simulink model "CF018A_GmRoadWhlInQlfr"  (R2013b)
settings: Solver=FixedStepDiscrete  SolverMode=SingleTasking  StartTime=0.0  StopTime=1  FixedStep=0.002  RelTol=1e-3
values from neighbouring files (symbols this model uses):
  DELTAPLSROLLOVR_CNT_S16 = DataDict.Constant    [CF018A_GmRoadWhlInQlfr_DataDict.m]
  DELTATISTAMPCNTROLLOVR_CNT_S32 = DataDict.Constant    [CF018A_GmRoadWhlInQlfr_DataDict.m]
  GmRoadWhlInQlfrMaxAllwblFrq = DataDict.Calibration    [CF018A_GmRoadWhlInQlfr_DataDict.m]
  GmRoadWhlInQlfrMaxFrqChg = DataDict.Calibration    [CF018A_GmRoadWhlInQlfr_DataDict.m]
  LEFRQCHGOUTOFRNG_CNT_U08 = DataDict.Constant    [CF018A_GmRoadWhlInQlfr_DataDict.m]
  LEFRQOUTOFRNG_CNT_U08 = DataDict.Constant    [CF018A_GmRoadWhlInQlfr_DataDict.m]
  NODEBSTEP_CNT_U16 = DataDict.Constant    [CF018A_GmRoadWhlInQlfr_DataDict.m]
  PARKDURN_CNT_F32 = DataDict.Constant    [CF018A_GmRoadWhlInQlfr_DataDict.m]
  PREVRAWWHLFRQMIN_HZ_F32 = DataDict.Constant    [CF018A_GmRoadWhlInQlfr_DataDict.m]
  RIFRQCHGOUTOFRNG_CNT_U08 = DataDict.Constant    [CF018A_GmRoadWhlInQlfr_DataDict.m]
  RIFRQOUTOFRNG_CNT_U08 = DataDict.Constant    [CF018A_GmRoadWhlInQlfr_DataDict.m]
  SECTO100MICROSECCNVN_CNT_F32 = DataDict.Constant    [CF018A_GmRoadWhlInQlfr_DataDict.m]
  WHLFRQMIN_HZ_F32 = DataDict.Constant    [CF018A_GmRoadWhlInQlfr_DataDict.m]
undefined symbols (not defined in the file or in its folder): NtcNr1, NtcSts1
libraries: simulink x8, NxtrAbslt x2, NxtrLim x2
(part 2 of 5)

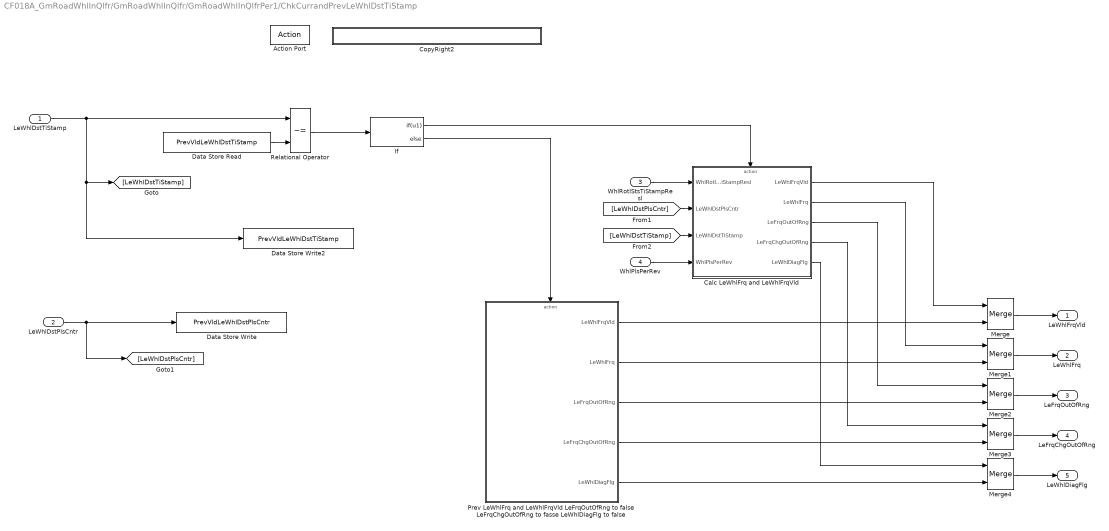
== system CF018A_GmRoadWhlInQlfr/GmRoadWhlInQlfr/GmRoadWhlInQlfrPer1/ChkCurrandPrevLeWhlDstTiStamp ==
  LeWhlDstTiStamp : Inport  RequirementInfo="{'linktype_rmi_doors' '0000c6e7 (/GM T1XX/SubSystem Specifications/Customer Functions/CF018A GM Road Wheel Input Qualifier)' '#174' 'true' 'REQ:  174' '' ; 'linktype_rmi_doors' '0000c6e7 (/GM T1XX/SubSystem Specifications/Customer Functions/CF018A GM Road Wheel Input Qualifier)' '#172' 'true' 'REQ:  172' '' ; 'linktype_rmi_doors' '0000c6e7 (/GM T1XX/SubSystem Specifications/Customer Functions/CF018A GM Road Wheel Input Qualifier)' '#172' 'true' 'REQ:  172' '' } %GIDa_1edc5147_117f_466a_8f92_e1f300aba7a4"
  LeWhlDstPlsCntr : Inport  RequirementInfo="{'linktype_rmi_doors' '0000c6e7 (/GM T1XX/SubSystem Specifications/Customer Functions/CF018A GM Road Wheel Input Qualifier)' '#174' 'true' 'REQ:  174' '' ; 'linktype_rmi_doors' '0000c6e7 (/GM T1XX/SubSystem Specifications/Customer Functions/CF018A GM Road Wheel Input Qualifier)' '#172' 'true' 'REQ:  172' '' } %GIDa_599ac311_8a22_418b_b4e0_03b5bb744075"  Port=2
  WhlRotlStsTiStampResl : Inport  RequirementInfo="{'linktype_rmi_doors' '0000c6e7 (/GM T1XX/SubSystem Specifications/Customer Functions/CF018A GM Road Wheel Input Qualifier)' '#172' 'true' 'REQ:  172' '' } %GIDa_a6510751_6b9d_4ed4_a7a9_c0455e316efd"  Port=3
  WhlPlsPerRev : Inport  RequirementInfo="{'linktype_rmi_doors' '0000c6e7 (/GM T1XX/SubSystem Specifications/Customer Functions/CF018A GM Road Wheel Input Qualifier)' '#172' 'true' 'REQ:  172' '' } %GIDa_b7be02b7_11d7_40a6_809e_b2017e30a38a"  Port=4
  Action Port : ActionPort  ActionType=else
  "Calc LeWhlFrq and LeWhlFrqVld " : Subsystem  RequirementInfo="{'linktype_rmi_doors' '0000c6e7 (/GM T1XX/SubSystem Specifications/Customer Functions/CF018A GM Road Wheel Input Qualifier)' '#172' 'true' 'REQ:  172' '' } %GIDa_4f3dc1f5_4afb_4260_bb3a_586610af36fa"  TreatAsAtomicUnit=on
      settings: AttributesFormatString=%<Priority>
  CopyRight2 : Subsystem  Description=|  mask(Copyright Information){none=on}
      | Copyright info block.                                               
      |                                                                     
      | Place copyright information at the top of every subsystem in design.
      mask prompts: none "No parameters"
      mask help: Place copyright information at the top of every subsystem in design.
      mask Display:
      | NxtrConf = 'Nexteer Confidential';
      | 
      | sys = bdroot; %handle for the current model ("system")
      | first = get_param(sys,'Created');
      | if(isempty(first))
      |     first = datestr(now,'yyyy');
      | else
      |     first = first(end-3:end);  %year is last four digits
      | end
      | 
      | last = get_param(sys,'LastModifiedDate');
      | if isempty(last)
      |     last = datestr(now,'yyyy');
      | else
      |     last = last(end-3:end);
      | end
      | 
      | if strcmp(first,last)
      |     fprintf('%s -- Copyright %s Nexteer',NxtrConf,first)
      | else
      |     fprintf('%s -- %s%s- %s Nexteer',NxtrConf,char(169),first,last)
      | end
  Data Store Read : DataStoreRead  RequirementInfo="{'linktype_rmi_doors' '0000c6e7 (/GM T1XX/SubSystem Specifications/Customer Functions/CF018A GM Road Wheel Input Qualifier)' '#174' 'true' 'REQ:  174' '' ; 'linktype_rmi_doors' '0000c6e7 (/GM T1XX/SubSystem Specifications/Customer Functions/CF018A GM Road Wheel Input Qualifier)' '#172' 'true' 'REQ:  172' '' ; 'linktype_rmi_doors' '0000c6e7 (/GM T1XX/SubSystem Specifications/Customer Functions/CF018A GM Road Wheel Input Qualifier)' '#172' 'true' 'REQ:  172' '' } %GIDa_b02de942_6a04_4580_afa9_b3288210702f"  Priority=0  DataStoreName=PrevVldLeWhlDstTiStamp
      settings: AttributesFormatString=%<Priority>
  Data Store Write : DataStoreWrite  RequirementInfo="{'linktype_rmi_doors' '0000c6e7 (/GM T1XX/SubSystem Specifications/Customer Functions/CF018A GM Road Wheel Input Qualifier)' '#174' 'true' 'REQ:  174' '' ; 'linktype_rmi_doors' '0000c6e7 (/GM T1XX/SubSystem Specifications/Customer Functions/CF018A GM Road Wheel Input Qualifier)' '#172' 'true' 'REQ:  172' '' } %GIDa_a502ae3f_c815_4164_88b0_c5b442c65c19"  Priority=2  DataStoreName=PrevVldLeWhlDstPlsCntr
      settings: AttributesFormatString=%<Priority>
  Data Store Write2 : DataStoreWrite  RequirementInfo="{'linktype_rmi_doors' '0000c6e7 (/GM T1XX/SubSystem Specifications/Customer Functions/CF018A GM Road Wheel Input Qualifier)' '#174' 'true' 'REQ:  174' '' ; 'linktype_rmi_doors' '0000c6e7 (/GM T1XX/SubSystem Specifications/Customer Functions/CF018A GM Road Wheel Input Qualifier)' '#172' 'true' 'REQ:  172' '' } %GIDa_ece9e0a0_953f_437a_8e6e_b4cc8c21fda4"  Priority=2  DataStoreName=PrevVldLeWhlDstTiStamp
      settings: AttributesFormatString=%<Priority>
  If : If  RequirementInfo="{'linktype_rmi_doors' '0000c6e7 (/GM T1XX/SubSystem Specifications/Customer Functions/CF018A GM Road Wheel Input Qualifier)' '#174' 'true' 'REQ:  174' '' ; 'linktype_rmi_doors' '0000c6e7 (/GM T1XX/SubSystem Specifications/Customer Functions/CF018A GM Road Wheel Input Qualifier)' '#172' 'true' 'REQ:  172' '' ; 'linktype_rmi_doors' '0000c6e7 (/GM T1XX/SubSystem Specifications/Customer Functions/CF018A GM Road Wheel Input Qualifier)' '#172' 'true' 'REQ:  172' '' } %GIDa_623ca339_0f35_4816_a941_00824c8527d2"  Priority=1  IfExpression=u1
      settings: AttributesFormatString=%<Priority>
  Merge{,1..4} (5 alike) : Merge
  "Prev LeWhlFrq and LeWhlFrqVld LeFrqOutOfRng to false LeFrqChgOutOfRng to fasse LeWhlDiagFlg to false " : Subsystem  RequirementInfo="{'linktype_rmi_doors' '0000c6e7 (/GM T1XX/SubSystem Specifications/Customer Functions/CF018A GM Road Wheel Input Qualifier)' '#174' 'true' 'REQ:  174' '' } %GIDa_5ebd6336_ff2e_47bd_9598_9199716c73c5"  TreatAsAtomicUnit=on
  Relational Operator : RelationalOperator  RequirementInfo="{'linktype_rmi_doors' '0000c6e7 (/GM T1XX/SubSystem Specifications/Customer Functions/CF018A GM Road Wheel Input Qualifier)' '#174' 'true' 'REQ:  174' '' ; 'linktype_rmi_doors' '0000c6e7 (/GM T1XX/SubSystem Specifications/Customer Functions/CF018A GM Road Wheel Input Qualifier)' '#172' 'true' 'REQ:  172' '' ; 'linktype_rmi_doors' '0000c6e7 (/GM T1XX/SubSystem Specifications/Customer Functions/CF018A GM Road Wheel Input Qualifier)' '#172' 'true' 'REQ:  172' '' } %GIDa_87ebce60_f387_4632_9316_04e7de82df91"  Operator=~=  OutDataTypeStr=boolean
  LeWhlFrqVld : Outport
  LeWhlFrq : Outport  Port=2
  LeFrqOutOfRng : Outport  Port=3
  LeFrqChgOutOfRng : Outport  Port=4
  LeWhlDiagFlg : Outport  Port=5
  wires:
  If/1 -> "Calc LeWhlFrq and LeWhlFrqVld "/Action
  WhlRotlStsTiStampResl/1 -> "Calc LeWhlFrq and LeWhlFrqVld "/1(WhlRotlStsTiStampResl)
  LeWhlDstPlsCntr/1 -> Data Store Write/1, [LeWhlDstPlsCntr]
  [LeWhlDstPlsCntr] -> "Calc LeWhlFrq and LeWhlFrqVld "/2(LeWhlDstPlsCntr)
  [LeWhlDstTiStamp] -> "Calc LeWhlFrq and LeWhlFrqVld "/3(LeWhlDstTiStamp)
  WhlPlsPerRev/1 -> "Calc LeWhlFrq and LeWhlFrqVld "/4(WhlPlsPerRev)
  Relational Operator/1 -> If/1
  Data Store Read/1 -> Relational Operator/2
  LeWhlDstTiStamp/1 -> Relational Operator/1, Data Store Write2/1, [LeWhlDstTiStamp]
  If/2 -> "Prev LeWhlFrq and LeWhlFrqVld LeFrqOutOfRng to false LeFrqChgOutOfRng to fasse LeWhlDiagFlg to false "/Action
  "Prev LeWhlFrq and LeWhlFrqVld LeFrqOutOfRng to false LeFrqChgOutOfRng to fasse LeWhlDiagFlg to false "/4(LeFrqChgOutOfRng) -> Merge3/2
  "Prev LeWhlFrq and LeWhlFrqVld LeFrqOutOfRng to false LeFrqChgOutOfRng to fasse LeWhlDiagFlg to false "/3(LeFrqOutOfRng) -> Merge2/2
  "Prev LeWhlFrq and LeWhlFrqVld LeFrqOutOfRng to false LeFrqChgOutOfRng to fasse LeWhlDiagFlg to false "/2(LeWhlFrq) -> Merge1/2
  "Prev LeWhlFrq and LeWhlFrqVld LeFrqOutOfRng to false LeFrqChgOutOfRng to fasse LeWhlDiagFlg to false "/1(LeWhlFrqVld) -> Merge/2
  "Calc LeWhlFrq and LeWhlFrqVld "/1(LeWhlFrqVld) -> Merge/1
  "Calc LeWhlFrq and LeWhlFrqVld "/2(LeWhlFrq) -> Merge1/1
  "Calc LeWhlFrq and LeWhlFrqVld "/3(LeFrqOutOfRng) -> Merge2/1
  "Calc LeWhlFrq and LeWhlFrqVld "/4(LeFrqChgOutOfRng) -> Merge3/1
  Merge/1 -> LeWhlFrqVld/1
  Merge1/1 -> LeWhlFrq/1
  Merge2/1 -> LeFrqOutOfRng/1
  Merge3/1 -> LeFrqChgOutOfRng/1
  "Calc LeWhlFrq and LeWhlFrqVld "/5(LeWhlDiagFlg) -> Merge4/1
  "Prev LeWhlFrq and LeWhlFrqVld LeFrqOutOfRng to false LeFrqChgOutOfRng to fasse LeWhlDiagFlg to false "/5(LeWhlDiagFlg) -> Merge4/2
  Merge4/1 -> LeWhlDiagFlg/1

== system CF018A_GmRoadWhlInQlfr/GmRoadWhlInQlfr/GmRoadWhlInQlfrPer1/CopyRight2 ==

== system CF018A_GmRoadWhlInQlfr/GmRoadWhlInQlfr/GmRoadWhlInQlfrPer1/NTC Diag ==
  LeFrqOutOfRng : Inport  RequirementInfo="{'linktype_rmi_doors' '0000c6e7 (/GM T1XX/SubSystem Specifications/Customer Functions/CF018A GM Road Wheel Input Qualifier)' '#53' 'true' 'REQ:  53' '' } %GIDa_bae70605_31ad_47de_93e2_34b5a485cde8"
  LeFrqChgOutOfRng : Inport  RequirementInfo="{'linktype_rmi_doors' '0000c6e7 (/GM T1XX/SubSystem Specifications/Customer Functions/CF018A GM Road Wheel Input Qualifier)' '#53' 'true' 'REQ:  53' '' } %GIDa_e1b25c35_a3b3_48ae_865c_0be9f62ee40d"  Port=2
  RiFrqOutOfRng : Inport  RequirementInfo="{'linktype_rmi_doors' '0000c6e7 (/GM T1XX/SubSystem Specifications/Customer Functions/CF018A GM Road Wheel Input Qualifier)' '#53' 'true' 'REQ:  53' '' } %GIDa_31ff7ea8_be27_4839_9d0c_e89098cdec37"  Port=3
  RiFrqChgOutOfRng : Inport  RequirementInfo="{'linktype_rmi_doors' '0000c6e7 (/GM T1XX/SubSystem Specifications/Customer Functions/CF018A GM Road Wheel Input Qualifier)' '#53' 'true' 'REQ:  53' '' } %GIDa_d26123b2_819a_4208_b0a7_2d9f46403555"  Port=4
  Action Port : ActionPort  ActionType=then
  Constant7 : Constant  RequirementInfo="{'linktype_rmi_doors' '0000c6e7 (/GM T1XX/SubSystem Specifications/Customer Functions/CF018A GM Road Wheel Input Qualifier)' '#53' 'true' 'REQ:  53' '' } %GIDa_40ab3d2e_6992_4126_9d67_b6070ef67c87"  Value=NODEBSTEP_CNT_U16
  Constant8 : Constant  RequirementInfo="{'linktype_rmi_doors' '0000c6e7 (/GM T1XX/SubSystem Specifications/Customer Functions/CF018A GM Road Wheel Input Qualifier)' '#53' 'true' 'REQ:  53' '' } %GIDa_77dfdcf3_e931_43d1_8caf_f6541dba129c"  Value=0  OutDataTypeStr=uint8
  Enumerated Constant2 : simulink/Sources/Enumerated Constant  RequirementInfo="{'linktype_rmi_doors' '0000c6e7 (/GM T1XX/SubSystem Specifications/Customer Functions/CF018A GM Road Wheel Input Qualifier)' '#53' 'true' 'REQ:  53' '' } %GIDa_ff40414a_bc98_44c9_a836_28923ef7b0e2"  OutDataTypeStr=Enum: NtcNr1  Value=NtcNr1.NTCNR_0X0E3  SampleTime=inf
  Enumerated Constant3 : simulink/Sources/Enumerated Constant  RequirementInfo="{'linktype_rmi_doors' '0000c6e7 (/GM T1XX/SubSystem Specifications/Customer Functions/CF018A GM Road Wheel Input Qualifier)' '#53' 'true' 'REQ:  53' '' } %GIDa_cfcf815d_81ef_4798_a053_4d41e7c75542"  OutDataTypeStr=Enum: NtcSts1  Value=NtcSts1.NTCSTS_PASSD  SampleTime=inf
  If2 : If  RequirementInfo="{'linktype_rmi_doors' '0000c6e7 (/GM T1XX/SubSystem Specifications/Customer Functions/CF018A GM Road Wheel Input Qualifier)' '#53' 'true' 'REQ:  53' '' } %GIDa_3353ee46_94e0_40a5_b784_e082bbbbc02d"  IfExpression=u1
  Logical Operator : Logic  RequirementInfo="{'linktype_rmi_doors' '0000c6e7 (/GM T1XX/SubSystem Specifications/Customer Functions/CF018A GM Road Wheel Input Qualifier)' '#53' 'true' 'REQ:  53' '' } %GIDa_fa2d2b95_4496_42fd_8f91_86f1fb2eadd8"  Operator=OR  Inputs=4  AllPortsSameDT=off  OutDataTypeStr=boolean
  NTC 0x0E3 Faild : Subsystem  RequirementInfo="{'linktype_rmi_doors' '0000c6e7 (/GM T1XX/SubSystem Specifications/Customer Functions/CF018A GM Road Wheel Input Qualifier)' '#53' 'true' 'REQ:  53' '' } %GIDa_49e1fe86_dba3_482d_9812_54f10c7cfaaf"  TreatAsAtomicUnit=on
  NTC 0x0E3 Passd : Subsystem  RequirementInfo="{'linktype_rmi_doors' '0000c6e7 (/GM T1XX/SubSystem Specifications/Customer Functions/CF018A GM Road Wheel Input Qualifier)' '#53' 'true' 'REQ:  53' '' } %GIDa_3990bfa5_7e5f_4316_8018_426f321c385b"  mask(SetNTC){}
      mask help: SetNTC library block
  wires:
  Logical Operator/1 -> If2/1
  If2/1 -> NTC 0x0E3 Faild/Action
  If2/2 -> NTC 0x0E3 Passd/Action
  Enumerated Constant2/1 -> NTC 0x0E3 Passd/1(NtcNr)
  Enumerated Constant3/1 -> NTC 0x0E3 Passd/3(NtcSts)
  Constant7/1 -> NTC 0x0E3 Passd/4(DebStep)
  Constant8/1 -> NTC 0x0E3 Passd/2(NtcStInfo)
  LeFrqOutOfRng/1 -> NTC 0x0E3 Faild/1(LeFrqOutOfRng), Logical Operator/1
  LeFrqChgOutOfRng/1 -> NTC 0x0E3 Faild/2(LeFrqChgOutOfRng), Logical Operator/2
  RiFrqOutOfRng/1 -> NTC 0x0E3 Faild/3(RiFrqOutOfRng), Logical Operator/3
  RiFrqChgOutOfRng/1 -> NTC 0x0E3 Faild/4(RiFrqChgOutOfRng), Logical Operator/4

== system CF018A_GmRoadWhlInQlfr/GmRoadWhlInQlfr/GmRoadWhlInQlfrPer1/Set Min Le whl Frq and false  ==
  Action Port : ActionPort  ActionType=then
  Constant1 : Constant  Value=WHLFRQMIN_HZ_F32  OutDataTypeStr=single
  Constant2 : Constant  Value=false  OutDataTypeStr=boolean
      settings: AttributesFormatString=%<OutDataTypeStr>
  CopyRight2 : Subsystem  Description=|  mask(Copyright Information){none=on}
      | Copyright info block.                                               
      |                                                                     
      | Place copyright information at the top of every subsystem in design.
      mask prompts: none "No parameters"
      mask help: Place copyright information at the top of every subsystem in design.
      mask Display:
      | NxtrConf = 'Nexteer Confidential';
      | 
      | sys = bdroot; %handle for the current model ("system")
      | first = get_param(sys,'Created');
      | if(isempty(first))
      |     first = datestr(now,'yyyy');
      | else
      |     first = first(end-3:end);  %year is last four digits
      | end
      | 
      | last = get_param(sys,'LastModifiedDate');
      | if isempty(last)
      |     last = datestr(now,'yyyy');
      | else
      |     last = last(end-3:end);
      | end
      | 
      | if strcmp(first,last)
      |     fprintf('%s -- Copyright %s Nexteer',NxtrConf,first)
      | else
      |     fprintf('%s -- %s%s- %s Nexteer',NxtrConf,char(169),first,last)
      | end
  LeWhlFrqVld : Outport
  LeWhlFrq : Outport  Port=2
  wires:
  Constant1/1 -> LeWhlFrq/1
  Constant2/1 -> LeWhlFrqVld/1

== system CF018A_GmRoadWhlInQlfr/GmRoadWhlInQlfr/GmRoadWhlInQlfrPer1/Set Min Ri whl Frq and false  ==
  Action Port : ActionPort  ActionType=then
  Constant1 : Constant  Value=WHLFRQMIN_HZ_F32  OutDataTypeStr=single
  Constant2 : Constant  Value=false  OutDataTypeStr=boolean
      settings: AttributesFormatString=%<OutDataTypeStr>
  CopyRight2 : Subsystem  Description=|  mask(Copyright Information){none=on}
      | Copyright info block.                                               
      |                                                                     
      | Place copyright information at the top of every subsystem in design.
      mask prompts: none "No parameters"
      mask help: Place copyright information at the top of every subsystem in design.
      mask Display:
      | NxtrConf = 'Nexteer Confidential';
      | 
      | sys = bdroot; %handle for the current model ("system")
      | first = get_param(sys,'Created');
      | if(isempty(first))
      |     first = datestr(now,'yyyy');
      | else
      |     first = first(end-3:end);  %year is last four digits
      | end
      | 
      | last = get_param(sys,'LastModifiedDate');
      | if isempty(last)
      |     last = datestr(now,'yyyy');
      | else
      |     last = last(end-3:end);
      | end
      | 
      | if strcmp(first,last)
      |     fprintf('%s -- Copyright %s Nexteer',NxtrConf,first)
      | else
      |     fprintf('%s -- %s%s- %s Nexteer',NxtrConf,char(169),first,last)
      | end
  RiWhlFrqVld : Outport
  RiWhlFrq : Outport  Port=2
  wires:
  Constant2/1 -> RiWhlFrqVld/1
  Constant1/1 -> RiWhlFrq/1

== system CF018A_GmRoadWhlInQlfr/GmRoadWhlInQlfr/GmRoadWhlInQlfrInit1/NTC 0x0E3 Passd/SetNtcSts ==
  NtcNr : Inport
  NtcStInfo : Inport  Port=2
  NtcSts : Inport  Port=3
  DebStep : Inport  Port=4
  CopyRight2 : Subsystem  Description=|  mask(Copyright Information){none=on}
      | Copyright info block.                                               
      |                                                                     
      | Place copyright information at the top of every subsystem in design.
      mask prompts: none "No parameters"
      mask help: Place copyright information at the top of every subsystem in design.
      mask Display:
      | NxtrConf = 'Nexteer Confidential';
      | 
      | sys = bdroot; %handle for the current model ("system")
      | first = get_param(sys,'Created');
      | first = first(end-3:end);  %year is last four digits
      | 
      | last = get_param(sys,'LastModifiedDate');
      | if isempty(last)
      |     last = datestr(now,'yyyy');
      | else
      |     last = last(end-3:end);
      | end
      | 
      | if strcmp(first,last)
      |     fprintf('%s -- Copyright %s Nexteer',NxtrConf,first)
      | else
      |     fprintf('%s -- %s%s- %s Nexteer',NxtrConf,char(169),first,last)
      | end
  Data Store Write3 : DataStoreWrite  DataStoreName=RoadWhlFrqInCalcOutOfRng
  Terminator : Terminator
  Terminator1 : Terminator
  Terminator2 : Terminator
  wires:
  DebStep/1 -> Terminator2/1
  NtcSts/1 -> Data Store Write3/1
  NtcNr/1 -> Terminator/1
  NtcStInfo/1 -> Terminator1/1

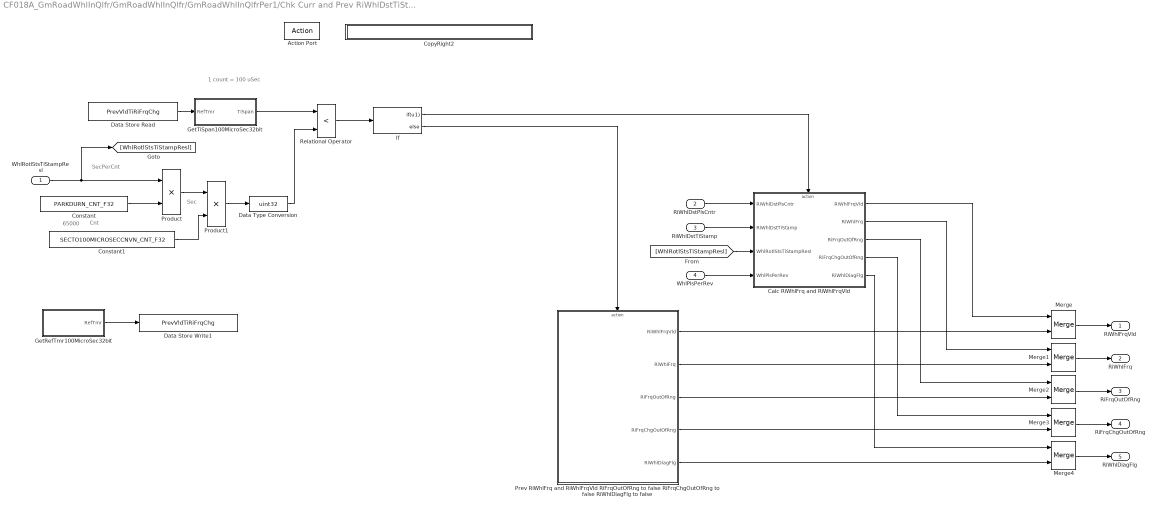
== system CF018A_GmRoadWhlInQlfr/GmRoadWhlInQlfr/GmRoadWhlInQlfrPer1/Chk Curr and Prev RiWhlDstTiStamp/Calc RiWhlFrq and RiWhlFrqVld  ==
  note: 1 count = 100 uSec
  note: SecPerCnt
  note: Cnt
  note: Sec
  note: 65000
  WhlRotlStsTiStampResl : Inport  RequirementInfo="{'linktype_rmi_doors' '0000c6e7 (/GM T1XX/SubSystem Specifications/Customer Functions/CF018A GM Road Wheel Input Qualifier)' '#193' 'true' 'REQ:  193' '' } %GIDa_b1960aa9_0c44_4de4_8b54_eab327ac46df"
  RiWhlDstPlsCntr : Inport  RequirementInfo="{'linktype_rmi_doors' '0000c6e7 (/GM T1XX/SubSystem Specifications/Customer Functions/CF018A GM Road Wheel Input Qualifier)' '#193' 'true' 'REQ:  193' '' } %GIDa_620ce4e7_830b_4e68_bf07_f05982ae0af3"  Port=2
  RiWhlDstTiStamp : Inport  RequirementInfo="{'linktype_rmi_doors' '0000c6e7 (/GM T1XX/SubSystem Specifications/Customer Functions/CF018A GM Road Wheel Input Qualifier)' '#193' 'true' 'REQ:  193' '' } %GIDa_cd0517c5_a032_4589_8c8a_e71bba42cf8d"  Port=3
  WhlPlsPerRev : Inport  RequirementInfo="{'linktype_rmi_doors' '0000c6e7 (/GM T1XX/SubSystem Specifications/Customer Functions/CF018A GM Road Wheel Input Qualifier)' '#193' 'true' 'REQ:  193' '' } %GIDa_7b76d69c_588c_4e8c_836d_0bbc914cccd7"  Port=4
  Action Port : ActionPort  ActionType=then
  "Calc RiWhlFrq and RiWhlFrqVld " : Subsystem  RequirementInfo="{'linktype_rmi_doors' '0000c6e7 (/GM T1XX/SubSystem Specifications/Customer Functions/CF018A GM Road Wheel Input Qualifier)' '#193' 'true' 'REQ:  193' '' } %GIDa_11737143_606c_4cac_b7b8_5b7d8549d8e9"  TreatAsAtomicUnit=on
  Constant : Constant  RequirementInfo="{'linktype_rmi_doors' '0000c6e7 (/GM T1XX/SubSystem Specifications/Customer Functions/CF018A GM Road Wheel Input Qualifier)' '#193' 'true' 'REQ:  193' '' } %GIDa_fc60505b_4e8b_4519_ba82_e46be79d957f"  Value=PARKDURN_CNT_F32  OutDataTypeStr=single
  Constant1 : Constant  RequirementInfo="{'linktype_rmi_doors' '0000c6e7 (/GM T1XX/SubSystem Specifications/Customer Functions/CF018A GM Road Wheel Input Qualifier)' '#193' 'true' 'REQ:  193' '' } %GIDa_e507e8ae_501a_4c72_a4c0_8e3ae5e945e5"  Value=SECTO100MICROSECCNVN_CNT_F32  OutDataTypeStr=single
  CopyRight2 : Subsystem  Description=|  mask(Copyright Information){none=on}
      | Copyright info block.                                               
      |                                                                     
      | Place copyright information at the top of every subsystem in design.
      mask prompts: none "No parameters"
      mask help: Place copyright information at the top of every subsystem in design.
      mask Display:
      | NxtrConf = 'Nexteer Confidential';
      | 
      | sys = bdroot; %handle for the current model ("system")
      | first = get_param(sys,'Created');
      | if(isempty(first))
      |     first = datestr(now,'yyyy');
      | else
      |     first = first(end-3:end);  %year is last four digits
      | end
      | 
      | last = get_param(sys,'LastModifiedDate');
      | if isempty(last)
      |     last = datestr(now,'yyyy');
      | else
      |     last = last(end-3:end);
      | end
      | 
      | if strcmp(first,last)
      |     fprintf('%s -- Copyright %s Nexteer',NxtrConf,first)
      | else
      |     fprintf('%s -- %s%s- %s Nexteer',NxtrConf,char(169),first,last)
      | end
  Data Store Read : DataStoreRead  RequirementInfo="{'linktype_rmi_doors' '0000c6e7 (/GM T1XX/SubSystem Specifications/Customer Functions/CF018A GM Road Wheel Input Qualifier)' '#193' 'true' 'REQ:  193' '' } %GIDa_06dfef7d_e885_4c7b_9844_561267c316d2"  Priority=0  DataStoreName=PrevVldTiRiFrqChg
      settings: AttributesFormatString=%<Priority>
  Data Store Write1 : DataStoreWrite  RequirementInfo="{'linktype_rmi_doors' '0000c6e7 (/GM T1XX/SubSystem Specifications/Customer Functions/CF018A GM Road Wheel Input Qualifier)' '#193' 'true' 'REQ:  193' '' } %GIDa_295187a8_a2d4_4e22_a32a_63e111fb6589"  Priority=1  DataStoreName=PrevVldTiRiFrqChg
      settings: AttributesFormatString=%<Priority>
  Data Type Conversion : DataTypeConversion  RequirementInfo="{'linktype_rmi_doors' '0000c6e7 (/GM T1XX/SubSystem Specifications/Customer Functions/CF018A GM Road Wheel Input Qualifier)' '#193' 'true' 'REQ:  193' '' } %GIDa_69165870_dfcd_405d_b7b0_09aaa14e44db"  OutDataTypeStr=uint32
  GetRefTmr100MicroSec32bit : Subsystem  RequirementInfo="{'linktype_rmi_doors' '0000c6e7 (/GM T1XX/SubSystem Specifications/Customer Functions/CF018A GM Road Wheel Input Qualifier)' '#193' 'true' 'REQ:  193' '' } %GIDa_c9e36b9e_70ac_4a04_a164_8d3115d80f8e"
  GetTiSpan100MicroSec32bit : Subsystem  RequirementInfo="{'linktype_rmi_doors' '0000c6e7 (/GM T1XX/SubSystem Specifications/Customer Functions/CF018A GM Road Wheel Input Qualifier)' '#193' 'true' 'REQ:  193' '' } %GIDa_497d2a53_795f_466e_9ad7_e72e9f51e5e0"
  If : If  RequirementInfo="{'linktype_rmi_doors' '0000c6e7 (/GM T1XX/SubSystem Specifications/Customer Functions/CF018A GM Road Wheel Input Qualifier)' '#193' 'true' 'REQ:  193' '' } %GIDa_295973ce_0db4_49ed_a178_a8fa4afac980"  IfExpression=u1
  Merge : Merge  RequirementInfo="{'linktype_rmi_doors' '0000c6e7 (/GM T1XX/SubSystem Specifications/Customer Functions/CF018A GM Road Wheel Input Qualifier)' '#193' 'true' 'REQ:  193' '' } %GIDa_c88d8626_0058_42c7_af05_4f446daff33c"
  Merge1 : Merge  RequirementInfo="{'linktype_rmi_doors' '0000c6e7 (/GM T1XX/SubSystem Specifications/Customer Functions/CF018A GM Road Wheel Input Qualifier)' '#193' 'true' 'REQ:  193' '' } %GIDa_895a51c6_5c33_4d42_9f4b_5ff8a415d996"
  Merge2 : Merge  RequirementInfo="{'linktype_rmi_doors' '0000c6e7 (/GM T1XX/SubSystem Specifications/Customer Functions/CF018A GM Road Wheel Input Qualifier)' '#193' 'true' 'REQ:  193' '' } %GIDa_29840dca_92c3_4d9f_b249_ad8260612163"
  Merge3 : Merge  RequirementInfo="{'linktype_rmi_doors' '0000c6e7 (/GM T1XX/SubSystem Specifications/Customer Functions/CF018A GM Road Wheel Input Qualifier)' '#193' 'true' 'REQ:  193' '' } %GIDa_b91213de_0f4e_48d0_8635_c0dc38d4c3c3"
  Merge4 : Merge  RequirementInfo="{'linktype_rmi_doors' '0000c6e7 (/GM T1XX/SubSystem Specifications/Customer Functions/CF018A GM Road Wheel Input Qualifier)' '#193' 'true' 'REQ:  193' '' } %GIDa_1b08c545_a32c_4e06_b0d0_0614948daffa"
  "Prev RiWhlFrq and RiWhlFrqVld RiFrqOutOfRng to false RiFrqChgOutOfRng to false RiWhlDiagFlg to false " : Subsystem  RequirementInfo="{'linktype_rmi_doors' '0000c6e7 (/GM T1XX/SubSystem Specifications/Customer Functions/CF018A GM Road Wheel Input Qualifier)' '#193' 'true' 'REQ:  193' '' } %GIDa_4ae01eac_d363_4811_8605_6241914f434f"  TreatAsAtomicUnit=on
  Product : Product  RequirementInfo="{'linktype_rmi_doors' '0000c6e7 (/GM T1XX/SubSystem Specifications/Customer Functions/CF018A GM Road Wheel Input Qualifier)' '#193' 'true' 'REQ:  193' '' } %GIDa_4c766cd3_1b27_4dcc_9920_41d79286be24"
  Product1 : Product  RequirementInfo="{'linktype_rmi_doors' '0000c6e7 (/GM T1XX/SubSystem Specifications/Customer Functions/CF018A GM Road Wheel Input Qualifier)' '#193' 'true' 'REQ:  193' '' } %GIDa_5675dbcb_6842_4205_ada9_7ff0fa3c3506"
  Relational Operator : RelationalOperator  RequirementInfo="{'linktype_rmi_doors' '0000c6e7 (/GM T1XX/SubSystem Specifications/Customer Functions/CF018A GM Road Wheel Input Qualifier)' '#193' 'true' 'REQ:  193' '' } %GIDa_0b5651dc_56e2_4239_856f_13fdf05ac3b9"  Operator=<  OutDataTypeStr=boolean
  RiWhlFrqVld : Outport  RequirementInfo="{'linktype_rmi_doors' '0000c6e7 (/GM T1XX/SubSystem Specifications/Customer Functions/CF018A GM Road Wheel Input Qualifier)' '#193' 'true' 'REQ:  193' '' } %GIDa_4ccf45da_49b8_43c1_a7f8_b9addd2b2c61"
  RiWhlFrq : Outport  RequirementInfo="{'linktype_rmi_doors' '0000c6e7 (/GM T1XX/SubSystem Specifications/Customer Functions/CF018A GM Road Wheel Input Qualifier)' '#193' 'true' 'REQ:  193' '' } %GIDa_d4a351a5_39b5_4b63_85a1_f1473d2e28d4"  Port=2
  RiFrqOutOfRng : Outport  RequirementInfo="{'linktype_rmi_doors' '0000c6e7 (/GM T1XX/SubSystem Specifications/Customer Functions/CF018A GM Road Wheel Input Qualifier)' '#193' 'true' 'REQ:  193' '' } %GIDa_2ea1f4e3_caef_49c0_aca8_d6e30198b656"  Port=3
  RiFrqChgOutOfRng : Outport  RequirementInfo="{'linktype_rmi_doors' '0000c6e7 (/GM T1XX/SubSystem Specifications/Customer Functions/CF018A GM Road Wheel Input Qualifier)' '#193' 'true' 'REQ:  193' '' } %GIDa_c7d84343_c50a_431f_85ac_0cd861b26476"  Port=4
  RiWhlDiagFlg : Outport  RequirementInfo="{'linktype_rmi_doors' '0000c6e7 (/GM T1XX/SubSystem Specifications/Customer Functions/CF018A GM Road Wheel Input Qualifier)' '#193' 'true' 'REQ:  193' '' } %GIDa_5968d98a_0992_4204_94cb_00d39b08e65e"  Port=5
  wires:
  Product/1 -> Product1/1
  Product1/1 -> Data Type Conversion/1
  Constant1/1 -> Product1/2
  Data Store Read/1 -> GetTiSpan100MicroSec32bit/1(RefTmr)
  RiWhlDstTiStamp/1 -> "Calc RiWhlFrq and RiWhlFrqVld "/2(RiWhlDstTiStamp)
  RiWhlDstPlsCntr/1 -> "Calc RiWhlFrq and RiWhlFrqVld "/1(RiWhlDstPlsCntr)
  GetTiSpan100MicroSec32bit/1(TiSpan) -> Relational Operator/1
  WhlPlsPerRev/1 -> "Calc RiWhlFrq and RiWhlFrqVld "/4(WhlPlsPerRev)
  [WhlRotlStsTiStampResl] -> "Calc RiWhlFrq and RiWhlFrqVld "/3(WhlRotlStsTiStampResl)
  If/1 -> "Calc RiWhlFrq and RiWhlFrqVld "/Action
  Relational Operator/1 -> If/1
  Constant/1 -> Product/2
  GetRefTmr100MicroSec32bit/1(RefTmr) -> Data Store Write1/1
  WhlRotlStsTiStampResl/1 -> Product/1, [WhlRotlStsTiStampResl]
  Data Type Conversion/1 -> Relational Operator/2
  "Prev RiWhlFrq and RiWhlFrqVld RiFrqOutOfRng to false RiFrqChgOutOfRng to false RiWhlDiagFlg to false "/4(RiFrqChgOutOfRng) -> Merge3/2
  "Prev RiWhlFrq and RiWhlFrqVld RiFrqOutOfRng to false RiFrqChgOutOfRng to false RiWhlDiagFlg to false "/3(RiFrqOutOfRng) -> Merge2/2
  "Prev RiWhlFrq and RiWhlFrqVld RiFrqOutOfRng to false RiFrqChgOutOfRng to false RiWhlDiagFlg to false "/2(RiWhlFrq) -> Merge1/2
  Merge1/1 -> RiWhlFrq/1
  Merge2/1 -> RiFrqOutOfRng/1
  Merge3/1 -> RiFrqChgOutOfRng/1
  "Calc RiWhlFrq and RiWhlFrqVld "/2(RiWhlFrq) -> Merge1/1
  "Calc RiWhlFrq and RiWhlFrqVld "/1(RiWhlFrqVld) -> Merge/1
  "Prev RiWhlFrq and RiWhlFrqVld RiFrqOutOfRng to false RiFrqChgOutOfRng to false RiWhlDiagFlg to false "/1(RiWhlFrqVld) -> Merge/2
  "Calc RiWhlFrq and RiWhlFrqVld "/3(RiFrqOutOfRng) -> Merge2/1
  "Calc RiWhlFrq and RiWhlFrqVld "/4(RiFrqChgOutOfRng) -> Merge3/1
  Merge/1 -> RiWhlFrqVld/1
  If/2 -> "Prev RiWhlFrq and RiWhlFrqVld RiFrqOutOfRng to false RiFrqChgOutOfRng to false RiWhlDiagFlg to false "/Action
  "Calc RiWhlFrq and RiWhlFrqVld "/5(RiWhlDiagFlg) -> Merge4/1
  "Prev RiWhlFrq and RiWhlFrqVld RiFrqOutOfRng to false RiFrqChgOutOfRng to false RiWhlDiagFlg to false "/5(RiWhlDiagFlg) -> Merge4/2
  Merge4/1 -> RiWhlDiagFlg/1

== system CF018A_GmRoadWhlInQlfr/GmRoadWhlInQlfr/GmRoadWhlInQlfrPer1/Chk Curr and Prev RiWhlDstTiStamp/CopyRight2 ==

== system CF018A_GmRoadWhlInQlfr/GmRoadWhlInQlfr/GmRoadWhlInQlfrPer1/Chk Curr and Prev RiWhlDstTiStamp/Prev RiWhlFrq and RiWhlFrqVld RiFrqOutOfRng to false RiFrqChgOutOfRng to false RiWhlDiagFlg to false  ==
  Action Port : ActionPort  ActionType=else
  Constant1 : Constant  Value=false  OutDataTypeStr=boolean
      settings: AttributesFormatString=%<OutDataTypeStr>
  Constant2 : Constant  Value=false  OutDataTypeStr=boolean
      settings: AttributesFormatString=%<OutDataTypeStr>
  Constant3 : Constant  Value=false  OutDataTypeStr=boolean
      settings: AttributesFormatString=%<OutDataTypeStr>
  Data Store Read2 : DataStoreRead  DataStoreName=PrevRiWhlFrqVld
      settings: AttributesFormatString=%<Priority>
  Data Store Read3 : DataStoreRead  DataStoreName=PrevRiWhlFrq
      settings: AttributesFormatString=%<Priority>
  RiWhlFrqVld : Outport
  RiWhlFrq : Outport  Port=2
  RiFrqOutOfRng : Outport  Port=3
  RiFrqChgOutOfRng : Outport  Port=4
  RiWhlDiagFlg : Outport  Port=5
  wires:
  Data Store Read2/1 -> RiWhlFrqVld/1
  Data Store Read3/1 -> RiWhlFrq/1
  Constant1/1 -> RiFrqOutOfRng/1
  Constant2/1 -> RiFrqChgOutOfRng/1
  Constant3/1 -> RiWhlDiagFlg/1

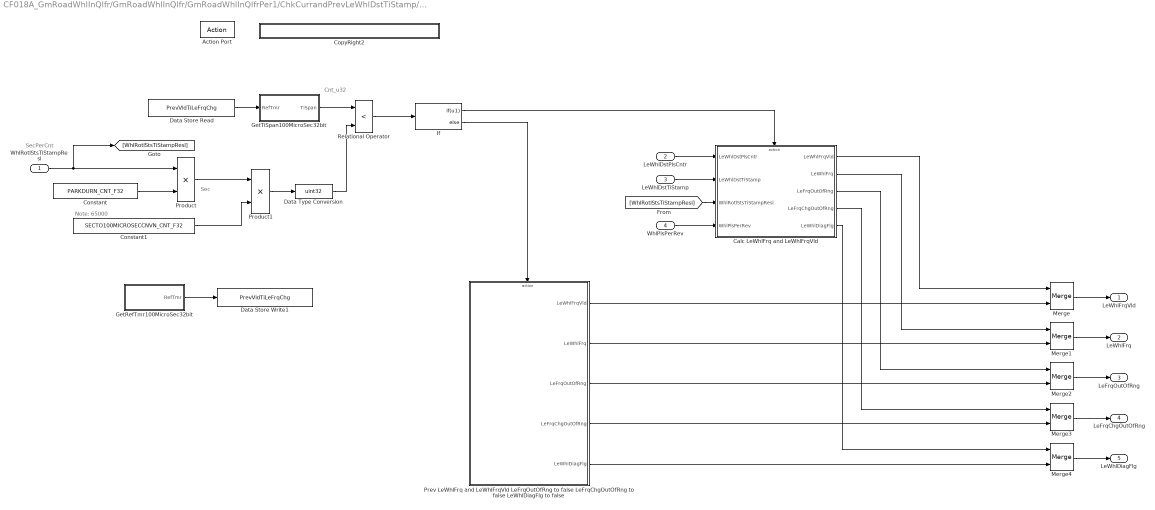
== system CF018A_GmRoadWhlInQlfr/GmRoadWhlInQlfr/GmRoadWhlInQlfrPer1/ChkCurrandPrevLeWhlDstTiStamp/Calc LeWhlFrq and LeWhlFrqVld  ==
  note: Cnt_u32
  note: Note: 65000
  note: Sec
  note: SecPerCnt
  WhlRotlStsTiStampResl : Inport  RequirementInfo="{'linktype_rmi_doors' '0000c6e7 (/GM T1XX/SubSystem Specifications/Customer Functions/CF018A GM Road Wheel Input Qualifier)' '#170' 'true' 'REQ:  170' '' } %GIDa_dd451c7e_a35d_45d7_832d_0f295eef8b4e"
  LeWhlDstPlsCntr : Inport  RequirementInfo="{'linktype_rmi_doors' '0000c6e7 (/GM T1XX/SubSystem Specifications/Customer Functions/CF018A GM Road Wheel Input Qualifier)' '#170' 'true' 'REQ:  170' '' } %GIDa_63dec2c8_8f26_46b5_b813_83b5d52f7513"  Port=2
  LeWhlDstTiStamp : Inport  RequirementInfo="{'linktype_rmi_doors' '0000c6e7 (/GM T1XX/SubSystem Specifications/Customer Functions/CF018A GM Road Wheel Input Qualifier)' '#170' 'true' 'REQ:  170' '' } %GIDa_d74960ce_6883_481a_900b_3939fe4e241c"  Port=3
  WhlPlsPerRev : Inport  RequirementInfo="{'linktype_rmi_doors' '0000c6e7 (/GM T1XX/SubSystem Specifications/Customer Functions/CF018A GM Road Wheel Input Qualifier)' '#170' 'true' 'REQ:  170' '' } %GIDa_3a27648a_5017_47e8_aff0_0afa4196b83f"  Port=4
  Action Port : ActionPort  ActionType=then
  "Calc LeWhlFrq and LeWhlFrqVld " : Subsystem  RequirementInfo="{'linktype_rmi_doors' '0000c6e7 (/GM T1XX/SubSystem Specifications/Customer Functions/CF018A GM Road Wheel Input Qualifier)' '#170' 'true' 'REQ:  170' '' } %GIDa_5ba6983e_9598_4595_9c3c_6d95ce34649c"  TreatAsAtomicUnit=on
  Constant : Constant  RequirementInfo="{'linktype_rmi_doors' '0000c6e7 (/GM T1XX/SubSystem Specifications/Customer Functions/CF018A GM Road Wheel Input Qualifier)' '#170' 'true' 'REQ:  170' '' } %GIDa_f88dce8d_fe82_4aa8_95bc_27d45b3b7387"  Value=PARKDURN_CNT_F32  OutDataTypeStr=single
  Constant1 : Constant  RequirementInfo="{'linktype_rmi_doors' '0000c6e7 (/GM T1XX/SubSystem Specifications/Customer Functions/CF018A GM Road Wheel Input Qualifier)' '#170' 'true' 'REQ:  170' '' } %GIDa_767294a5_1ea7_420a_b1a9_e4131c82f064"  Value=SECTO100MICROSECCNVN_CNT_F32  OutDataTypeStr=single
  CopyRight2 : Subsystem  Description=|  mask(Copyright Information){none=on}
      | Copyright info block.                                               
      |                                                                     
      | Place copyright information at the top of every subsystem in design.
      mask prompts: none "No parameters"
      mask help: Place copyright information at the top of every subsystem in design.
      mask Display:
      | NxtrConf = 'Nexteer Confidential';
      | 
      | sys = bdroot; %handle for the current model ("system")
      | first = get_param(sys,'Created');
      | if(isempty(first))
      |     first = datestr(now,'yyyy');
      | else
      |     first = first(end-3:end);  %year is last four digits
      | end
      | 
      | last = get_param(sys,'LastModifiedDate');
      | if isempty(last)
      |     last = datestr(now,'yyyy');
      | else
      |     last = last(end-3:end);
      | end
      | 
      | if strcmp(first,last)
      |     fprintf('%s -- Copyright %s Nexteer',NxtrConf,first)
      | else
      |     fprintf('%s -- %s%s- %s Nexteer',NxtrConf,char(169),first,last)
      | end
  Data Store Read : DataStoreRead  RequirementInfo="{'linktype_rmi_doors' '0000c6e7 (/GM T1XX/SubSystem Specifications/Customer Functions/CF018A GM Road Wheel Input Qualifier)' '#170' 'true' 'REQ:  170' '' } %GIDa_e311223d_6aad_44ed_8afb_0e69877d0ed9"  Priority=0  DataStoreName=PrevVldTiLeFrqChg
      settings: AttributesFormatString=%<Priority>
  Data Store Write1 : DataStoreWrite  RequirementInfo="{'linktype_rmi_doors' '0000c6e7 (/GM T1XX/SubSystem Specifications/Customer Functions/CF018A GM Road Wheel Input Qualifier)' '#170' 'true' 'REQ:  170' '' } %GIDa_026fa113_0cb7_4ff3_94d7_8176222ac909"  Priority=1  DataStoreName=PrevVldTiLeFrqChg
      settings: AttributesFormatString=%<Priority>
  Data Type Conversion : DataTypeConversion  RequirementInfo="{'linktype_rmi_doors' '0000c6e7 (/GM T1XX/SubSystem Specifications/Customer Functions/CF018A GM Road Wheel Input Qualifier)' '#170' 'true' 'REQ:  170' '' } %GIDa_30be5bf4_1952_4a5b_a980_01a868b94654"  OutDataTypeStr=uint32
  GetRefTmr100MicroSec32bit : Subsystem  RequirementInfo="{'linktype_rmi_doors' '0000c6e7 (/GM T1XX/SubSystem Specifications/Customer Functions/CF018A GM Road Wheel Input Qualifier)' '#170' 'true' 'REQ:  170' '' } %GIDa_7d9c4050_4b52_4184_9390_b52e07327fa8"
  GetTiSpan100MicroSec32bit : Subsystem  RequirementInfo="{'linktype_rmi_doors' '0000c6e7 (/GM T1XX/SubSystem Specifications/Customer Functions/CF018A GM Road Wheel Input Qualifier)' '#170' 'true' 'REQ:  170' '' } %GIDa_2b1b068f_100b_4c76_9b29_5a84168298e0"
  If : If  RequirementInfo="{'linktype_rmi_doors' '0000c6e7 (/GM T1XX/SubSystem Specifications/Customer Functions/CF018A GM Road Wheel Input Qualifier)' '#170' 'true' 'REQ:  170' '' } %GIDa_2eba1a84_5614_4bc6_b732_13cc45ab6882"  IfExpression=u1
  Merge : Merge  RequirementInfo="{'linktype_rmi_doors' '0000c6e7 (/GM T1XX/SubSystem Specifications/Customer Functions/CF018A GM Road Wheel Input Qualifier)' '#170' 'true' 'REQ:  170' '' } %GIDa_41cda46e_0ed0_4ffc_a2bf_159c5af030fd"
  Merge1 : Merge  RequirementInfo="{'linktype_rmi_doors' '0000c6e7 (/GM T1XX/SubSystem Specifications/Customer Functions/CF018A GM Road Wheel Input Qualifier)' '#170' 'true' 'REQ:  170' '' } %GIDa_07cb30f9_4463_4be1_8de1_3df8af68cb8e"
  Merge2 : Merge  RequirementInfo="{'linktype_rmi_doors' '0000c6e7 (/GM T1XX/SubSystem Specifications/Customer Functions/CF018A GM Road Wheel Input Qualifier)' '#170' 'true' 'REQ:  170' '' } %GIDa_82e8ed07_da74_41a4_8eee_fb68b8956ea1"
  Merge3 : Merge  RequirementInfo="{'linktype_rmi_doors' '0000c6e7 (/GM T1XX/SubSystem Specifications/Customer Functions/CF018A GM Road Wheel Input Qualifier)' '#170' 'true' 'REQ:  170' '' } %GIDa_74b9fe88_d24c_4841_9553_38d2025a47be"
  Merge4 : Merge  RequirementInfo="{'linktype_rmi_doors' '0000c6e7 (/GM T1XX/SubSystem Specifications/Customer Functions/CF018A GM Road Wheel Input Qualifier)' '#170' 'true' 'REQ:  170' '' } %GIDa_a72ceeb0_adb2_4102_ac2d_a2b17625ca57"
  "Prev LeWhlFrq and LeWhlFrqVld LeFrqOutOfRng to false LeFrqChgOutOfRng to false LeWhlDiagFlg to false " : Subsystem  RequirementInfo="{'linktype_rmi_doors' '0000c6e7 (/GM T1XX/SubSystem Specifications/Customer Functions/CF018A GM Road Wheel Input Qualifier)' '#170' 'true' 'REQ:  170' '' } %GIDa_e5b8e4ff_4db3_4ac3_aae7_d3637005cb4e"  TreatAsAtomicUnit=on
  Product : Product  RequirementInfo="{'linktype_rmi_doors' '0000c6e7 (/GM T1XX/SubSystem Specifications/Customer Functions/CF018A GM Road Wheel Input Qualifier)' '#170' 'true' 'REQ:  170' '' } %GIDa_e22cf699_f626_44b9_9342_8ac55b23899d"  OutDataTypeStr=single
  Product1 : Product  RequirementInfo="{'linktype_rmi_doors' '0000c6e7 (/GM T1XX/SubSystem Specifications/Customer Functions/CF018A GM Road Wheel Input Qualifier)' '#170' 'true' 'REQ:  170' '' } %GIDa_ddb6dcf6_3805_46d3_b31b_f2246b796a82"
  Relational Operator : RelationalOperator  RequirementInfo="{'linktype_rmi_doors' '0000c6e7 (/GM T1XX/SubSystem Specifications/Customer Functions/CF018A GM Road Wheel Input Qualifier)' '#170' 'true' 'REQ:  170' '' } %GIDa_daa8bf2f_2e0b_4156_918d_aa8d3c9b2125"  Operator=<  OutDataTypeStr=boolean
  LeWhlFrqVld : Outport  RequirementInfo="{'linktype_rmi_doors' '0000c6e7 (/GM T1XX/SubSystem Specifications/Customer Functions/CF018A GM Road Wheel Input Qualifier)' '#170' 'true' 'REQ:  170' '' } %GIDa_e5473e16_87d4_4d22_a1ce_c3c3311bfddb"
  LeWhlFrq : Outport  RequirementInfo="{'linktype_rmi_doors' '0000c6e7 (/GM T1XX/SubSystem Specifications/Customer Functions/CF018A GM Road Wheel Input Qualifier)' '#170' 'true' 'REQ:  170' '' } %GIDa_f2eed787_da2e_4295_b74c_710419094b16"  Port=2
  LeFrqOutOfRng : Outport  RequirementInfo="{'linktype_rmi_doors' '0000c6e7 (/GM T1XX/SubSystem Specifications/Customer Functions/CF018A GM Road Wheel Input Qualifier)' '#170' 'true' 'REQ:  170' '' } %GIDa_cc6c97e9_8ef1_42c0_9c54_056cfe415380"  Port=3
  LeFrqChgOutOfRng : Outport  RequirementInfo="{'linktype_rmi_doors' '0000c6e7 (/GM T1XX/SubSystem Specifications/Customer Functions/CF018A GM Road Wheel Input Qualifier)' '#170' 'true' 'REQ:  170' '' } %GIDa_daedcf58_9203_4373_854d_3d9fb367dfb4"  Port=4
  LeWhlDiagFlg : Outport  RequirementInfo="{'linktype_rmi_doors' '0000c6e7 (/GM T1XX/SubSystem Specifications/Customer Functions/CF018A GM Road Wheel Input Qualifier)' '#170' 'true' 'REQ:  170' '' } %GIDa_b2db63f7_5f7b_41cf_a04f_2f3d718b32a2"  Port=5
  wires:
  Constant/1 -> Product/2
  Relational Operator/1 -> If/1
  If/1 -> "Calc LeWhlFrq and LeWhlFrqVld "/Action
  [WhlRotlStsTiStampResl] -> "Calc LeWhlFrq and LeWhlFrqVld "/3(WhlRotlStsTiStampResl)
  WhlPlsPerRev/1 -> "Calc LeWhlFrq and LeWhlFrqVld "/4(WhlPlsPerRev)
  LeWhlDstPlsCntr/1 -> "Calc LeWhlFrq and LeWhlFrqVld "/1(LeWhlDstPlsCntr)
  LeWhlDstTiStamp/1 -> "Calc LeWhlFrq and LeWhlFrqVld "/2(LeWhlDstTiStamp)
  Constant1/1 -> Product1/2
  GetTiSpan100MicroSec32bit/1(TiSpan) -> Relational Operator/1
  GetRefTmr100MicroSec32bit/1(RefTmr) -> Data Store Write1/1
  Data Store Read/1 -> GetTiSpan100MicroSec32bit/1(RefTmr)
  WhlRotlStsTiStampResl/1 -> Product/1, [WhlRotlStsTiStampResl]
  Product/1 -> Product1/1
  Data Type Conversion/1 -> Relational Operator/2
  Product1/1 -> Data Type Conversion/1
  If/2 -> "Prev LeWhlFrq and LeWhlFrqVld LeFrqOutOfRng to false LeFrqChgOutOfRng to false LeWhlDiagFlg to false "/Action
  Merge/1 -> LeWhlFrqVld/1
  Merge1/1 -> LeWhlFrq/1
  Merge2/1 -> LeFrqOutOfRng/1
  Merge3/1 -> LeFrqChgOutOfRng/1
  "Calc LeWhlFrq and LeWhlFrqVld "/1(LeWhlFrqVld) -> Merge/1
  "Prev LeWhlFrq and LeWhlFrqVld LeFrqOutOfRng to false LeFrqChgOutOfRng to false LeWhlDiagFlg to false "/3(LeFrqOutOfRng) -> Merge2/2
  "Prev LeWhlFrq and LeWhlFrqVld LeFrqOutOfRng to false LeFrqChgOutOfRng to false LeWhlDiagFlg to false "/4(LeFrqChgOutOfRng) -> Merge3/2
  "Prev LeWhlFrq and LeWhlFrqVld LeFrqOutOfRng to false LeFrqChgOutOfRng to false LeWhlDiagFlg to false "/1(LeWhlFrqVld) -> Merge/2
  "Prev LeWhlFrq and LeWhlFrqVld LeFrqOutOfRng to false LeFrqChgOutOfRng to false LeWhlDiagFlg to false "/2(LeWhlFrq) -> Merge1/2
  "Calc LeWhlFrq and LeWhlFrqVld "/2(LeWhlFrq) -> Merge1/1
  "Calc LeWhlFrq and LeWhlFrqVld "/3(LeFrqOutOfRng) -> Merge2/1
  "Calc LeWhlFrq and LeWhlFrqVld "/4(LeFrqChgOutOfRng) -> Merge3/1
  "Calc LeWhlFrq and LeWhlFrqVld "/5(LeWhlDiagFlg) -> Merge4/1
  "Prev LeWhlFrq and LeWhlFrqVld LeFrqOutOfRng to false LeFrqChgOutOfRng to false LeWhlDiagFlg to false "/5(LeWhlDiagFlg) -> Merge4/2
  Merge4/1 -> LeWhlDiagFlg/1

== system CF018A_GmRoadWhlInQlfr/GmRoadWhlInQlfr/GmRoadWhlInQlfrPer1/ChkCurrandPrevLeWhlDstTiStamp/CopyRight2 ==

== system CF018A_GmRoadWhlInQlfr/GmRoadWhlInQlfr/GmRoadWhlInQlfrPer1/ChkCurrandPrevLeWhlDstTiStamp/Prev LeWhlFrq and LeWhlFrqVld LeFrqOutOfRng to false LeFrqChgOutOfRng to fasse LeWhlDiagFlg to false  ==
  Action Port : ActionPort  ActionType=else
  Constant1 : Constant  Value=false  OutDataTypeStr=boolean
      settings: AttributesFormatString=%<OutDataTypeStr>
  Constant2 : Constant  Value=false  OutDataTypeStr=boolean
      settings: AttributesFormatString=%<OutDataTypeStr>
  Constant3 : Constant  Value=false  OutDataTypeStr=boolean
      settings: AttributesFormatString=%<OutDataTypeStr>
  Data Store Read2 : DataStoreRead  DataStoreName=PrevLeWhlFrqVld
      settings: AttributesFormatString=%<Priority>
  Data Store Read3 : DataStoreRead  DataStoreName=PrevLeWhlFrq
      settings: AttributesFormatString=%<Priority>
  LeWhlFrqVld : Outport
  LeWhlFrq : Outport  Port=2
  LeFrqOutOfRng : Outport  Port=3
  LeFrqChgOutOfRng : Outport  Port=4
  LeWhlDiagFlg : Outport  Port=5
  wires:
  Data Store Read2/1 -> LeWhlFrqVld/1
  Data Store Read3/1 -> LeWhlFrq/1
  Constant1/1 -> LeFrqOutOfRng/1
  Constant2/1 -> LeFrqChgOutOfRng/1
  Constant3/1 -> LeWhlDiagFlg/1
